simulink model "ee_converter_dcdc_llc"  (R2019b)
settings: Solver=VariableStepAuto  StartTime=0.0  StopTime=2e-3  RelTol=1e-3  AbsTol=1e-3  EnableMultiTasking=on
PreLoadFcn:
  | Vbus_nominal = 450;
  | Vbus_ripple = 10;
  | busRippleFrequency = 100;
  | Vout_nominal = 54;
  | Pout = 100;
  | Cr = 1.5e-8;
  | Lr = 2e-4;
  | Lm_theory = 2.5e-3;
  | n = 4.3;
  | transformerCoupling = 0.99;
  | Cout = 3e-5;
  | tdead = 3e-7;
  | fswfinal = [68.7 93.7]*1e3;
  | Vf = 0.6;
  | 
  | switchType = 1;
StopFcn:
  | ee_addSimlogTimeStamp(bdroot)
undefined symbols (not defined in the file or in its folder): diff
libraries: ee_lib x12, fl_lib x10, nesl_utility x6, simulink x4
(part 2 of 2)

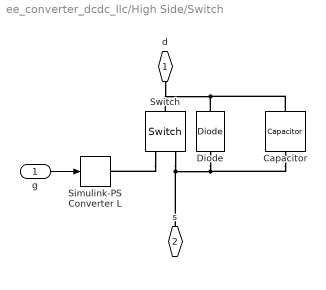
== system ee_converter_dcdc_llc/High Side/Switch ==
  g : Inport
  Capacitor : ee_lib/Passive/Capacitor  cap_option=1  c=14 pF  Cvec="[494  158  118  100   89   81   75   71   67   64   61   59   57   56   54   53   52   50   49   49   48   47   46   45   45   44   44   43   42   42   41   41   41   40   40   39   39   39   38   38   38   38   37   37   37   36   36   36   36   36 36] pF"  Vvec="[0   12   24   36   49   61   73   85   97  109  121  133  146  158  170  182  194  206  218  230  243  255  267  279  291  303  315  328  340  352  364  376  388  400  412  425  437  449  461  473  485  497  510  522  534  546  558  570  582  594 1000] V"  CV_table_symmetry=1  f_vec=[1, 10] kHz  DFext_vec=[.8, 1.2]  C_tol=5  enable_C_tol=0  tol_distribution=1  nSigma=4  r=1e-3 Ohm  g=1e-6 1/Ohm  averaging_period=0 s  enable_operating_limits=0  operating_limit_action=2  max_working_voltage_range=[ -25 25 ] V  power_rating=1 W  enable_faults=0  fault_action=1  Cscale_faulted=100  R_faulted=0.001 Ohm  G_faulted=0 1/Ohm  tau_fault=0.001 s  enable_temporal_fault=0  t_fault=1 s  enable_behavioral_fault=0  max_permissible_voltage_range=[ -100 100 ] V  t_fail_on_voltage=1 s  i_specify=off  i_priority=None  i=0 A  i_nominal_specify=off  i_nominal_unit=A  i_nominal_value=1  v_specify=off  v_priority=None  v=0 V  v_nominal_specify=off  v_nominal_unit=V  v_nominal_value=1  vc_specify=on  vc_priority=High  vc=Vbus_nominal V  vc_nominal_specify=off  vc_nominal_unit=V  vc_nominal_value=1
      settings: SourceProductName=Simscape Electrical
  Diode : fl_lib/Electrical/Electrical Elements/Diode  Vf=1.2 V  Ron=0.17 Ohm  Goff=1e-8 1/Ohm  i_specify=off  i_priority=None  i=0 A  i_nominal_specify=off  i_nominal_unit=A  i_nominal_value=1  v_specify=off  v_priority=None  v=0 V  v_nominal_specify=off  v_nominal_unit=V  v_nominal_value=1
  Simulink-PS Converter L : nesl_utility/Simulink-PS Converter  PhysicalDomain=network_engine_domain  SubClassName=ps_input  LeftPortType=input  RightPortType=output  PseudoPeriodic=off  Frequencies=[]  NoiseDistribution=none  NoiseParameters=[]  Unit=1  AffineConversion=off  FilteringAndDerivatives=zero  SimscapeFilterOrder=1  InputFilterTimeConstant=0.001  UdotUserProvided=1
  Switch : fl_lib/Electrical/Electrical Elements/Switch  R_closed=0.17 Ohm  G_open=1e-8 1/Ohm  Threshold=5  i_specify=off  i_priority=None  i=0 A  i_nominal_specify=off  i_nominal_unit=A  i_nominal_value=1  v_specify=off  v_priority=None  v=0 V  v_nominal_specify=off  v_nominal_unit=V  v_nominal_value=1
      settings: SourceProductName=Simscape
  d : PMIOPort  Side=Right
  s : PMIOPort  Port=2  Side=Right
  wires:
  g/1 -> Simulink-PS Converter L/1
  connections:
  s/RConn1 -- Capacitor/RConn1 -- Diode/LConn1 -- Switch/RConn2
  Switch/LConn1 -- d/RConn1 -- Diode/RConn1 -- Capacitor/LConn1
  Switch/RConn1 -- Simulink-PS Converter L/RConn1

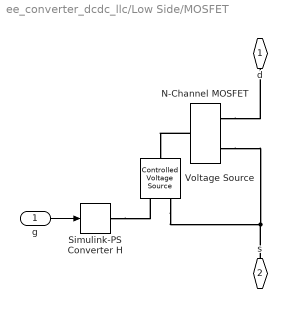
== system ee_converter_dcdc_llc/Low Side/MOSFET ==
  g : Inport
  N-Channel MOSFET : ee_lib/Semiconductors & Converters/N-Channel MOSFET  parameterization=1  prmDatasheet=1  prmEquCoeff=1  Beta=5.0 A/V^2  Rds=0.025 Ohm  Id=6.0 A  Vgs=10 V  Vth=1.7 V  lam=0 1/V  Tmeas=25 degC  RS=0.0001 Ohm  RD=0.01 Ohm  C_param=1  C_GS=270 pF  C_GD=80 pF  C_DS=0 pF  C_iss=350 pF  C_rss=80 pF  C_oss=0 pF  C_GS_vec=[270, 300, 290, 280, 295, 255] pF  C_GD_vec=[450, 400, 300, 190, 95, 55] pF  C_DS_vec=[450, 410, 390, 230, 175, 115] pF  C_iss_vec=[720, 700, 590, 470, 390, 310] pF  C_rss_vec=[450, 400, 300, 190, 95, 55] pF  C_oss_vec=[900, 810, 690, 420, 270, 170] pF  C_Vds_vec=[.1, .3, 1, 3, 10, 30] V  V_GS_for_cap_data=0 V  charge_linearity_param=1  C_OX=200 pF  V_C_OX=-0.5 V  IsDiode=0 A  Vbi=1.2 V  n=1  Cj0Diode=0 pF  TT=430 ns  dVth_dT=-6 mV/K  Rds_T2=0.037 Ohm  Tmeas2=125 degC  BEXDatasheet=-1.5  BEXEquCoeff=-1.5  etaisDatasheet=3  etaisEquCoeff=3  TdeviceDatasheet=25 degC  TdeviceEquCoeff=25 degC  thermal_network_parameterization=ee.enum.thermalNetworkTopology.cauer  Rth=[0, 10] K/W  Rth_Foster=[4, 6] K/W  thermal_mass_parameterization=ee.enum.thermalNetwork.timeconstant  thermal_mass=[0, 1] J/K  thermal_mass_Foster=[1.5, 3] J/K  thermal_time_constant=[0, 10] s  thermal_time_constant_Foster=[6, 18] s  thermal_mass_initial_temperatures=[25, 25] degC  betaref=18 A/V^2  Vfbref=- 1.1 V  gamma=3.5 V^0.50000  phib2ref=1 V  thesatref=0.4 1/V  alpha=0  Vp=5e-2 V  thesrref=0 1/V  m=2  Tref=298.15 K  Cox=1500 pF  Cgso=100 pF  Cgdo=14 pF  Rsref=2e-3 Ohm  Rdref=0.17 Ohm  Rgref=8.4 Ohm  Isref=5.2e-13 A  Cj0=480 pF  Tprm=1  etabet=1.3  Stvfb=5e-4 V/K  Stphib=- 8.5e-4 V/K  etasat=1.04  etasr=0.65  etar=0.95  etais=3  Tsim=298.15 K  T0=[25, 25] degC
      settings: SourceProductName=Simscape Electrical
  Simulink-PS Converter H : nesl_utility/Simulink-PS Converter  PhysicalDomain=network_engine_domain  SubClassName=ps_input  LeftPortType=input  RightPortType=output  PseudoPeriodic=off  Frequencies=[]  NoiseDistribution=none  NoiseParameters=[]  Unit=1  AffineConversion=off  FilteringAndDerivatives=zero  SimscapeFilterOrder=1  InputFilterTimeConstant=0.001  UdotUserProvided=1
  Voltage Source : fl_lib/Electrical/Electrical Sources/Controlled Voltage Source
  d : PMIOPort  Side=Right
  s : PMIOPort  Port=2  Side=Right
  wires:
  g/1 -> Simulink-PS Converter H/1
  connections:
  N-Channel MOSFET/RConn2 -- Voltage Source/RConn2 -- s/RConn1
  Simulink-PS Converter H/RConn1 -- Voltage Source/RConn1
  N-Channel MOSFET/LConn1 -- Voltage Source/LConn1
  N-Channel MOSFET/RConn1 -- d/RConn1

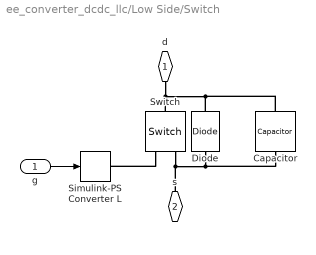
== system ee_converter_dcdc_llc/Low Side/Switch ==
  g : Inport
  Capacitor : ee_lib/Passive/Capacitor  cap_option=1  c=14 pF  Cvec="[494  158  118  100   89   81   75   71   67   64   61   59   57   56   54   53   52   50   49   49   48   47   46   45   45   44   44   43   42   42   41   41   41   40   40   39   39   39   38   38   38   38   37   37   37   36   36   36   36   36 36] pF"  Vvec="[0   12   24   36   49   61   73   85   97  109  121  133  146  158  170  182  194  206  218  230  243  255  267  279  291  303  315  328  340  352  364  376  388  400  412  425  437  449  461  473  485  497  510  522  534  546  558  570  582  594 1000] V"  CV_table_symmetry=1  f_vec=[1, 10] kHz  DFext_vec=[.8, 1.2]  C_tol=5  enable_C_tol=0  tol_distribution=1  nSigma=4  r=1e-3 Ohm  g=1e-6 1/Ohm  averaging_period=0 s  enable_operating_limits=0  operating_limit_action=2  max_working_voltage_range=[ -25 25 ] V  power_rating=1 W  enable_faults=0  fault_action=1  Cscale_faulted=100  R_faulted=0.001 Ohm  G_faulted=0 1/Ohm  tau_fault=0.001 s  enable_temporal_fault=0  t_fault=1 s  enable_behavioral_fault=0  max_permissible_voltage_range=[ -100 100 ] V  t_fail_on_voltage=1 s  i_specify=off  i_priority=None  i=0 A  i_nominal_specify=off  i_nominal_unit=A  i_nominal_value=1  v_specify=off  v_priority=None  v=0 V  v_nominal_specify=off  v_nominal_unit=V  v_nominal_value=1  vc_specify=on  vc_priority=High  vc=0 V  vc_nominal_specify=off  vc_nominal_unit=V  vc_nominal_value=1
      settings: SourceProductName=Simscape Electrical
  Diode : fl_lib/Electrical/Electrical Elements/Diode  Vf=1.2 V  Ron=0.17 Ohm  Goff=1e-8 1/Ohm  i_specify=off  i_priority=None  i=0 A  i_nominal_specify=off  i_nominal_unit=A  i_nominal_value=1  v_specify=off  v_priority=None  v=0 V  v_nominal_specify=off  v_nominal_unit=V  v_nominal_value=1
  Simulink-PS Converter L : nesl_utility/Simulink-PS Converter  PhysicalDomain=network_engine_domain  SubClassName=ps_input  LeftPortType=input  RightPortType=output  PseudoPeriodic=off  Frequencies=[]  NoiseDistribution=none  NoiseParameters=[]  Unit=1  AffineConversion=off  FilteringAndDerivatives=zero  SimscapeFilterOrder=1  InputFilterTimeConstant=0.001  UdotUserProvided=1
  Switch : fl_lib/Electrical/Electrical Elements/Switch  R_closed=0.17 Ohm  G_open=1e-8 1/Ohm  Threshold=5  i_specify=off  i_priority=None  i=0 A  i_nominal_specify=off  i_nominal_unit=A  i_nominal_value=1  v_specify=off  v_priority=None  v=0 V  v_nominal_specify=off  v_nominal_unit=V  v_nominal_value=1
      settings: SourceProductName=Simscape
  d : PMIOPort  Side=Right
  s : PMIOPort  Port=2  Side=Right
  wires:
  g/1 -> Simulink-PS Converter L/1
  connections:
  Switch/RConn1 -- Simulink-PS Converter L/RConn1
  d/RConn1 -- Switch/LConn1 -- Diode/RConn1 -- Capacitor/LConn1
  s/RConn1 -- Capacitor/RConn1 -- Diode/LConn1 -- Switch/RConn2

== system ee_converter_dcdc_llc/Behavioral Gate Driver/Gate Control Signals/Delayed-on high-side ==
  u : Inport
  Delayed logic : Logic  AllPortsSameDT=off  OutDataTypeStr=boolean
  One if tdead elapsed : Subsystem  TreatAsAtomicUnit=on
  y : Outport  VectorParamsAs1DForOutWhenUnconnected=off
  wires:
  u/1 -> Delayed logic/1, One if tdead elapsed/Enable
  One if tdead elapsed/1(y) -> Delayed logic/2
  Delayed logic/1 -> y/1

== system ee_converter_dcdc_llc/Behavioral Gate Driver/Gate Control Signals/Delayed-on low-side  ==
  u : Inport
  Delayed logic : Logic  AllPortsSameDT=off  OutDataTypeStr=boolean
  One if tdead elapsed : Subsystem  TreatAsAtomicUnit=on
  y : Outport  VectorParamsAs1DForOutWhenUnconnected=off
  wires:
  Delayed logic/1 -> y/1
  One if tdead elapsed/1(y) -> Delayed logic/2
  u/1 -> Delayed logic/1, One if tdead elapsed/Enable

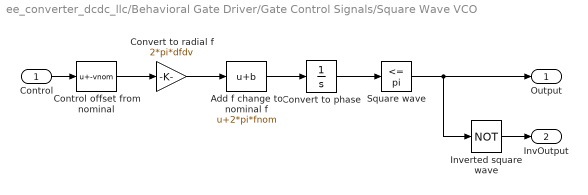
== system ee_converter_dcdc_llc/Behavioral Gate Driver/Gate Control Signals/Square Wave VCO ==
  Control : Inport
  Add f change to nominal f : Bias  Bias=2*pi*fnom
  Control offset from nominal : Bias  Bias=-vnom
  Convert to phase : Integrator  WrapState=on  WrappedStateUpperValue=2*pi  WrappedStateLowerValue=0
  Convert to radial f : Gain  Gain=2*pi*dfdv
  Inverted square wave : Logic  Operator=NOT  AllPortsSameDT=off  OutDataTypeStr=boolean
  Square wave : simulink/Logic and Bit Operations/Compare To Constant  relop=<=  const=pi  OutDataTypeStr=boolean
  Output : Outport  VectorParamsAs1DForOutWhenUnconnected=off
  InvOutput : Outport  Port=2  VectorParamsAs1DForOutWhenUnconnected=off
  wires:
  Convert to radial f/1 -> Add f change to nominal f/1
  Inverted square wave/1 -> InvOutput/1
  Square wave/1 -> Output/1, Inverted square wave/1
  Convert to phase/1 -> Square wave/1
  Control/1 -> Control offset from nominal/1
  Control offset from nominal/1 -> Convert to radial f/1
  Add f change to nominal f/1 -> Convert to phase/1

== system ee_converter_dcdc_llc/Behavioral Gate Driver/Gate Control Signals/Delayed-on high-side/One if tdead elapsed ==
  Enable : EnablePort  StatesWhenEnabling=reset
  Compare To Constant : simulink/Logic and Bit Operations/Compare To Constant  relop=>  const=tdead  OutDataTypeStr=boolean
  Constant : Constant
  Integrator : Integrator
  y : Outport  VectorParamsAs1DForOutWhenUnconnected=off
  wires:
  Constant/1 -> Integrator/1
  Integrator/1 -> Compare To Constant/1
  Compare To Constant/1 -> y/1

== system ee_converter_dcdc_llc/Behavioral Gate Driver/Gate Control Signals/Delayed-on low-side /One if tdead elapsed ==
  Enable : EnablePort  StatesWhenEnabling=reset
  Compare To Constant : simulink/Logic and Bit Operations/Compare To Constant  relop=>  const=tdead  OutDataTypeStr=boolean
  Constant : Constant
  Integrator : Integrator
  y : Outport  VectorParamsAs1DForOutWhenUnconnected=off
  wires:
  Compare To Constant/1 -> y/1
  Integrator/1 -> Compare To Constant/1
  Constant/1 -> Integrator/1
